simulink model "hip_controller_2026_02_23"  (R2024b)
settings: Solver=FixedStepAuto  StartTime=0.0  StopTime=simDuration  FixedStep=0.01  RelTol=1e-3  EnableMultiTasking=on
InitFcn:
  | breakp=[-1, -0.8, -0.6, -0.4, -0.2, -0.1, 0, 0.1, 0.2, 0.4, 0.6, 0.8, 1];
  | splinenew =[-1, -0.8, -0.6, -0.4, -0.2, -0.1, 0, 0, 0.005, 0.01, 0.015,0.02,0.025];
undefined symbols (not defined in the file or in its folder): Discrete, K, qbreak, Time
libraries: simulink x121, arduinolib x41, dspswit3 x21, ctrlSharedLib x2, dspfdesign x2, slpidlib x2
(part 3 of 7)

== system hip_controller_2026_02_23/Initialize Function/Config_R/Enter Config Mode ==
  Compare To Zero8 : simulink/Logic and Bit Operations/Compare To Zero  relop===  OutDataTypeStr=boolean
  Constant5 : Constant  Value=0x00
  Start_Config_R : arduinolib/I2C Write  I2CModule=0  Mode=Master  SlaveAddress=0x29  SlaveByteOrder=BigEndian  Direction=Transmitter  RegisterAddressMode=on  RegisterAddress=0x3D  SlaveDataType=uint8  DataLength=1  NoAck=off  RepeatedStart=off  OutputStatus=on  blockPlatform=ARDUINO
      settings: SourceProductName=Common
  Status : Outport
  wires:
  Start_Config_R/1 -> Compare To Zero8/1  "0 for success"
  Constant5/1 -> Start_Config_R/1
  Compare To Zero8/1 -> Status/1

== system hip_controller_2026_02_23/Initialize Function/Config_R/Start Fused (NDOF) Mode ==
  Enable : EnablePort
  Compare To Constant1 : simulink/Logic and Bit Operations/Compare To Constant  relop===  const=0  OutDataTypeStr=boolean
  Constant4 : Constant  Value=0x0C
  I2C Write8 : arduinolib/I2C Write  I2CModule=0  Mode=Master  SlaveAddress=0x29  SlaveByteOrder=BigEndian  Direction=Transmitter  RegisterAddressMode=on  RegisterAddress=0x3D  SlaveDataType=uint8  DataLength=1  NoAck=off  RepeatedStart=off  OutputStatus=on  blockPlatform=ARDUINO
      settings: SourceProductName=Common
  Status : Outport
  wires:
  Compare To Constant1/1 -> Status/1
  Constant4/1 -> I2C Write8/1
  I2C Write8/1 -> Compare To Constant1/1  "0: success"

== system hip_controller_2026_02_23/Initialize Function/Config_R/X=Z, Y=Y, Z=X ==
  Enable : EnablePort
  Compare To Constant : simulink/Logic and Bit Operations/Compare To Constant  relop=~=  const=hex2dec('06')  OutDataTypeStr=boolean
  Compare To Constant1 : simulink/Logic and Bit Operations/Compare To Constant  relop===  const=hex2dec('06')  OutDataTypeStr=boolean
  Enabled Subsystem : Subsystem  TreatAsAtomicUnit=on
  I2C Read : arduinolib/I2C Read  I2CModule=0  Mode=Master  SlaveAddress=0x29  SlaveByteOrder=LittleEndian  Direction=Receiver  RegisterAddressMode=on  RegisterAddress=0x41  SlaveDataType=uint8  DataLength=1  NoAck=off  RepeatedStart=off  OutputStatus=off  blockPlatform=ARDUINO  SampleTime=-1
      settings: SourceProductName=Common
  OR : Logic  Operator=OR  IconShape=distinctive  AllPortsSameDT=off  OutDataTypeStr=boolean
  Status : Outport
  wires:
  I2C Read/1 -> Compare To Constant1/1, Compare To Constant/1
  Compare To Constant1/1 -> OR/2
  Compare To Constant/1 -> Enabled Subsystem/Enable
  Enabled Subsystem/1(Status) -> OR/1
  OR/1 -> Status/1

== system hip_controller_2026_02_23/Initialize Function/Config_R/Z = -Z ==
  note: 0x01: Z = -Z
  Enable : EnablePort
  Compare To Constant : simulink/Logic and Bit Operations/Compare To Constant  relop=~=  const=hex2dec('01')  OutDataTypeStr=boolean
  Compare To Constant1 : simulink/Logic and Bit Operations/Compare To Constant  relop===  const=hex2dec('01')  OutDataTypeStr=boolean
  OR : Logic  Operator=OR  IconShape=distinctive  AllPortsSameDT=off  OutDataTypeStr=boolean
  Read : arduinolib/I2C Read  I2CModule=0  Mode=Master  SlaveAddress=0x29  SlaveByteOrder=LittleEndian  Direction=Receiver  RegisterAddressMode=on  RegisterAddress=0x42  SlaveDataType=uint8  DataLength=1  NoAck=off  RepeatedStart=off  OutputStatus=off  blockPlatform=ARDUINO  SampleTime=-1
      settings: SourceProductName=Common
  Write : Subsystem  TreatAsAtomicUnit=on
  Status : Outport
  wires:
  Write/1(Status) -> OR/1
  Compare To Constant/1 -> Write/Enable
  Read/1 -> Compare To Constant1/1, Compare To Constant/1
  Compare To Constant1/1 -> OR/2
  OR/1 -> Status/1

== system hip_controller_2026_02_23/LEFT LEG1/Pos and Vel normalized/Subsystem ==
  Angle : Inport
  Trigger : TriggerPort  VariantControl=Variant  PortDimensions=1
  Angle_min : Outport
  wires:
  Angle/1 -> Angle_min/1

== system hip_controller_2026_02_23/LEFT LEG1/Pos and Vel normalized/Subsystem1 ==
  Velocity : Inport
  Trigger : TriggerPort  VariantControl=Variant  PortDimensions=1
  Vel_max : Outport
  wires:
  Velocity/1 -> Vel_max/1

== system hip_controller_2026_02_23/LEFT LEG1/Pos and Vel normalized/Subsystem2 ==
  angle : Inport
  Trigger : TriggerPort  VariantControl=Variant  PortDimensions=1
  Angle_max : Outport
  wires:
  angle/1 -> Angle_max/1

== system hip_controller_2026_02_23/LEFT LEG1/Pos and Vel normalized/Subsystem3 ==
  Velocity : Inport
  Trigger : TriggerPort  VariantControl=Variant  PortDimensions=1
  Vel_min : Outport
  wires:
  Velocity/1 -> Vel_min/1

== system hip_controller_2026_02_23/LEFT LEG1/Pos and Vel normalized/Subsystem4 ==
  Clock : Inport
  angle : Inport  Port=2
  Trigger : TriggerPort  VariantControl=Variant  PortDimensions=1
  If : If  ShowElse=off
  If Action Subsystem : Subsystem  TreatAsAtomicUnit=on
  Angle_max : Outport
  wires:
  If/1 -> If Action Subsystem/Action
  angle/1 -> If Action Subsystem/2(angle), If/1
  If Action Subsystem/1(Angle_max) -> Angle_max/1  "angle_max"
  Clock/1 -> If Action Subsystem/1(Clock)  "clock"

== system hip_controller_2026_02_23/LEFT LEG1/Pos and Vel normalized/Subsystem5 ==
  Angle : Inport
  Clock : Inport  Port=2
  Trigger : TriggerPort  VariantControl=Variant  PortDimensions=1
  If : If  IfExpression=u1 < 0  ShowElse=off
  If Action Subsystem : Subsystem  TreatAsAtomicUnit=on
  Angle_min : Outport
  wires:
  If/1 -> If Action Subsystem/Action
  Angle/1 -> If Action Subsystem/1(Angle), If/1
  If Action Subsystem/1(Angle_min) -> Angle_min/1  "angle_min"
  Clock/1 -> If Action Subsystem/2(Clock)  "clock"

== system hip_controller_2026_02_23/LEFT LEG1/Pos and Vel normalized/Subsystem6 ==
  Velocity : Inport
  Clock : Inport  Port=2
  Trigger : TriggerPort  VariantControl=Variant  PortDimensions=1
  If : If  IfExpression=u1 < 0  ShowElse=off
  If Action Subsystem : Subsystem  TreatAsAtomicUnit=on
  Vel_min : Outport
  wires:
  If Action Subsystem/1(Vel_min) -> Vel_min/1  "vel_min"
  If/1 -> If Action Subsystem/Action
  Velocity/1 -> If Action Subsystem/1(Velocity), If/1
  Clock/1 -> If Action Subsystem/2(Clock)  "clock"

== system hip_controller_2026_02_23/LEFT LEG1/Pos and Vel normalized/Subsystem7 ==
  Velocity : Inport
  Clock : Inport  Port=2
  Trigger : TriggerPort  VariantControl=Variant  PortDimensions=1
  If : If  ShowElse=off
  If Action Subsystem : Subsystem  TreatAsAtomicUnit=on
  Vel_max : Outport
  wires:
  If/1 -> If Action Subsystem/Action
  Velocity/1 -> If Action Subsystem/1(Velocity), If/1
  Clock/1 -> If Action Subsystem/2(Clock)  "clock"
  If Action Subsystem/1(Vel_max) -> Vel_max/1  "vel_max"

== system hip_controller_2026_02_23/LEFT LEG3/GAIT PHASE BLOCK/CENTERING AND NORMALIZING ==
  Angle max : Inport
  Angle min : Inport  Port=2
  Vel max : Inport  Port=3
  Vel min : Inport  Port=4
  Trigger : TriggerPort  VariantControl=(inherit)  PortDimensions=1
  Abs : Abs  SaturateOnIntegerOverflow=off
  Abs1 : Abs  SaturateOnIntegerOverflow=off
  Constant : Constant  Value=0.5
  Constant1 : Constant  Value=0.5
  Divide : Product  Inputs=/*
  Product : Product
  Product1 : Product
  Sum : Sum
  Sum1 : Sum
  Sum2 : Sum  Inputs=+-
  Sum3 : Sum  Inputs=+-
  Switch : Switch  Criteria=u2 > Threshold  SaturateOnIntegerOverflow=off  InputSameDT=off
  Center vel : Outport
  Center angle : Outport  Port=2
  Gamma : Outport  Port=3
  wires:
  Divide/1 -> Gamma/1
  Abs1/1 -> Switch/3, Divide/2
  Switch/1 -> Divide/1
  Abs/1 -> Switch/1, Switch/2
  Sum3/1 -> Abs1/1
  Sum2/1 -> Abs/1
  Product1/1 -> Center vel/1
  Vel min/1 -> Sum1/2, Sum3/2
  Vel max/1 -> Sum1/1, Sum3/1
  Sum1/1 -> Product1/1
  Constant1/1 -> Product1/2
  Product/1 -> Center angle/1
  Constant/1 -> Product/2
  Sum/1 -> Product/1
  Angle min/1 -> Sum/2, Sum2/2
  Angle max/1 -> Sum/1, Sum2/1

== system hip_controller_2026_02_23/LEFT LEG3/GAIT PHASE BLOCK/LOGIC FOR THE BEGINNING ==
  Enable : EnablePort
  Constant : Constant  Value=0
  Phase to zero : Outport
  wires:
  Constant/1 -> Phase to zero/1

== system hip_controller_2026_02_23/LEFT LEG3/GAIT PHASE BLOCK/STRIDE EVENT DETECTOR ==
  In1 : Inport
  angle : Inport  Port=2
  Enable : EnablePort
  AND : Logic  IconShape=distinctive  AllPortsSameDT=off  OutDataTypeStr=boolean
  Hit Crossing5 : HitCross  HitCrossingOffset=-0.1  HitCrossingDirection=falling
  Relational Operator : RelationalOperator  OutDataTypeStr=boolean  RndMeth=Simplest  InputSameDT=off
  ~5 degrees : Constant  Value=0.08
  Out1 : Outport
  wires:
  Hit Crossing5/1 -> Out1/1
  ~5 degrees/1 -> Relational Operator/2
  Relational Operator/1 -> AND/2
  angle/1 -> Relational Operator/1
  In1/1 -> Hit Crossing5/1

== system hip_controller_2026_02_23/LEFT LEG3/GAIT PHASE BLOCK/Subsystem ==
  Input : Inport
  Trigger : TriggerPort  VariantControl=Variant  PortDimensions=1
  Angle min : Outport
  wires:
  Input/1 -> Angle min/1

== system hip_controller_2026_02_23/LEFT LEG3/GAIT PHASE BLOCK/Subsystem2 ==
  Input : Inport
  Trigger : TriggerPort  VariantControl=Variant  PortDimensions=1
  Angle max : Outport
  wires:
  Input/1 -> Angle max/1

== system hip_controller_2026_02_23/LEFT LEG3/GAIT PHASE BLOCK/Subsystem4 ==
  Input : Inport
  Trigger : TriggerPort  VariantControl=Variant  PortDimensions=1
  Vel min : Outport
  wires:
  Input/1 -> Vel min/1

== system hip_controller_2026_02_23/LEFT LEG3/GAIT PHASE BLOCK/Subsystem5 ==
  Input : Inport
  Trigger : TriggerPort  VariantControl=Variant  PortDimensions=1
  Vel max : Outport
  wires:
  Input/1 -> Vel max/1

== system hip_controller_2026_02_23/LEFT LEG3/Subsystem/SIGMOID SCALING ==
  note: a^n / (a^n + 1)
      |
      | The higher n, the more low amplitudes are scaled down
  PORTRAIT RADIUS : Inport
  Sigmoid Power : Inport  Port=2
  Constant2 : Constant
  Divide : Product  Inputs=*/
  Power : Math  Operator=pow
  Scale to 1 : Saturate  UpperLimit=1  LowerLimit=0
  Sum1 : Sum
  Out1 : Outport
  wires:
  Divide/1 -> Scale to 1/1
  PORTRAIT RADIUS/1 -> Power/1
  Power/1 -> Sum1/1, Divide/1
  Scale to 1/1 -> Out1/1
  Constant2/1 -> Sum1/2
  Sigmoid Power/1 -> Power/2  "sig_power_L"
  Sum1/1 -> Divide/2

== system hip_controller_2026_02_23/RIGHT LEG2/GAIT PHASE BLOCK/CENTERING AND NORMALIZING ==
  Angle max : Inport
  Angle min : Inport  Port=2
  Vel max : Inport  Port=3
  Vel min : Inport  Port=4
  Trigger : TriggerPort  VariantControl=(inherit)  PortDimensions=1
  Abs : Abs  SaturateOnIntegerOverflow=off
  Abs1 : Abs  SaturateOnIntegerOverflow=off
  Constant : Constant  Value=0.5
  Constant1 : Constant  Value=0.5
  Divide : Product  Inputs=/*
  Product : Product
  Product1 : Product
  Sum : Sum
  Sum1 : Sum
  Sum2 : Sum  Inputs=+-
  Sum3 : Sum  Inputs=+-
  Switch : Switch  Criteria=u2 > Threshold  SaturateOnIntegerOverflow=off  InputSameDT=off
  Center vel : Outport
  Center angle : Outport  Port=2
  Gamma : Outport  Port=3
  wires:
  Divide/1 -> Gamma/1
  Abs1/1 -> Switch/3, Divide/2
  Switch/1 -> Divide/1
  Abs/1 -> Switch/1, Switch/2
  Sum3/1 -> Abs1/1
  Sum2/1 -> Abs/1
  Product1/1 -> Center vel/1
  Vel min/1 -> Sum1/2, Sum3/2
  Vel max/1 -> Sum1/1, Sum3/1
  Sum1/1 -> Product1/1
  Constant1/1 -> Product1/2
  Product/1 -> Center angle/1
  Constant/1 -> Product/2
  Sum/1 -> Product/1
  Angle min/1 -> Sum/2, Sum2/2
  Angle max/1 -> Sum/1, Sum2/1

== system hip_controller_2026_02_23/RIGHT LEG2/GAIT PHASE BLOCK/LOGIC FOR THE BEGINNING ==
  Enable : EnablePort
  Constant : Constant  Value=0
  Phase to zero : Outport
  wires:
  Constant/1 -> Phase to zero/1

== system hip_controller_2026_02_23/RIGHT LEG2/GAIT PHASE BLOCK/STRIDE EVENT DETECTOR ==
  In1 : Inport
  angle : Inport  Port=2
  Enable : EnablePort
  AND : Logic  IconShape=distinctive  AllPortsSameDT=off  OutDataTypeStr=boolean
  Hit Crossing5 : HitCross  HitCrossingOffset=-0.1  HitCrossingDirection=falling
  Relational Operator : RelationalOperator  OutDataTypeStr=boolean  RndMeth=Simplest  InputSameDT=off
  ~5 degrees : Constant  Value=0.08
  Out1 : Outport
  wires:
  Hit Crossing5/1 -> Out1/1
  ~5 degrees/1 -> Relational Operator/2
  Relational Operator/1 -> AND/2
  angle/1 -> Relational Operator/1
  In1/1 -> Hit Crossing5/1

== system hip_controller_2026_02_23/RIGHT LEG2/GAIT PHASE BLOCK/Subsystem ==
  Input : Inport
  Trigger : TriggerPort  VariantControl=Variant  PortDimensions=1
  Angle min : Outport
  wires:
  Input/1 -> Angle min/1

== system hip_controller_2026_02_23/RIGHT LEG2/GAIT PHASE BLOCK/Subsystem2 ==
  Input : Inport
  Trigger : TriggerPort  VariantControl=Variant  PortDimensions=1
  Angle max : Outport
  wires:
  Input/1 -> Angle max/1

== system hip_controller_2026_02_23/RIGHT LEG2/GAIT PHASE BLOCK/Subsystem4 ==
  Input : Inport
  Trigger : TriggerPort  VariantControl=Variant  PortDimensions=1
  Vel min : Outport
  wires:
  Input/1 -> Vel min/1

== system hip_controller_2026_02_23/RIGHT LEG2/GAIT PHASE BLOCK/Subsystem5 ==
  Input : Inport
  Trigger : TriggerPort  VariantControl=Variant  PortDimensions=1
  Vel max : Outport
  wires:
  Input/1 -> Vel max/1

== system hip_controller_2026_02_23/RIGHT LEG2/Subsystem/SIGMOID SCALING ==
  note: a^n / (a^n + 1)
      |
      | The higher n, the more low amplitudes are scaled down
  PORTRAIT RADIUS : Inport
  sigmoid_power : Inport  Port=2
  Constant2 : Constant
  Divide : Product  Inputs=*/
  Power : Math  Operator=pow
  Scale to 1 : Saturate  UpperLimit=1  LowerLimit=0
  Sum1 : Sum
  Out1 : Outport
  wires:
  Divide/1 -> Scale to 1/1
  PORTRAIT RADIUS/1 -> Power/1
  Power/1 -> Sum1/1, Divide/1
  Scale to 1/1 -> Out1/1
  Constant2/1 -> Sum1/2
  sigmoid_power/1 -> Power/2
  Sum1/1 -> Divide/2

== system hip_controller_2026_02_23/RIGHT_LEG1/Pos and Vel normalized/Subsystem ==
  Angle : Inport
  Trigger : TriggerPort  VariantControl=Variant  PortDimensions=1
  Angle_min : Outport
  wires:
  Angle/1 -> Angle_min/1

== system hip_controller_2026_02_23/RIGHT_LEG1/Pos and Vel normalized/Subsystem1 ==
  Velocity : Inport
  Trigger : TriggerPort  VariantControl=Variant  PortDimensions=1
  Vel_max : Outport
  wires:
  Velocity/1 -> Vel_max/1

== system hip_controller_2026_02_23/RIGHT_LEG1/Pos and Vel normalized/Subsystem2 ==
  angle : Inport
  Trigger : TriggerPort  VariantControl=Variant  PortDimensions=1
  Angle_max : Outport
  wires:
  angle/1 -> Angle_max/1

== system hip_controller_2026_02_23/RIGHT_LEG1/Pos and Vel normalized/Subsystem3 ==
  Velocity : Inport
  Trigger : TriggerPort  VariantControl=Variant  PortDimensions=1
  Vel_min : Outport
  wires:
  Velocity/1 -> Vel_min/1

== system hip_controller_2026_02_23/RIGHT_LEG1/Pos and Vel normalized/Subsystem4 ==
  Clock : Inport
  angle : Inport  Port=2
  Trigger : TriggerPort  VariantControl=Variant  PortDimensions=1
  If : If  ShowElse=off
  If Action Subsystem : Subsystem  TreatAsAtomicUnit=on
  Angle_max : Outport
  wires:
  If/1 -> If Action Subsystem/Action
  angle/1 -> If Action Subsystem/2(angle), If/1
  If Action Subsystem/1(Angle_max) -> Angle_max/1  "angle_max"
  Clock/1 -> If Action Subsystem/1(Clock)  "clock"

== system hip_controller_2026_02_23/RIGHT_LEG1/Pos and Vel normalized/Subsystem5 ==
  Angle : Inport
  Clock : Inport  Port=2
  Trigger : TriggerPort  VariantControl=Variant  PortDimensions=1
  If : If  IfExpression=u1 < 0  ShowElse=off
  If Action Subsystem : Subsystem  TreatAsAtomicUnit=on
  Angle_min : Outport
  wires:
  If/1 -> If Action Subsystem/Action
  Angle/1 -> If Action Subsystem/1(Angle), If/1
  If Action Subsystem/1(Angle_min) -> Angle_min/1  "angle_min"
  Clock/1 -> If Action Subsystem/2(Clock)  "clock"

== system hip_controller_2026_02_23/RIGHT_LEG1/Pos and Vel normalized/Subsystem6 ==
  Velocity : Inport
  Clock : Inport  Port=2
  Trigger : TriggerPort  VariantControl=Variant  PortDimensions=1
  If : If  IfExpression=u1 < 0  ShowElse=off
  If Action Subsystem : Subsystem  TreatAsAtomicUnit=on
  Vel_min : Outport
  wires:
  If Action Subsystem/1(Vel_min) -> Vel_min/1  "vel_min"
  If/1 -> If Action Subsystem/Action
  Velocity/1 -> If Action Subsystem/1(Velocity), If/1
  Clock/1 -> If Action Subsystem/2(Clock)  "clock"

== system hip_controller_2026_02_23/RIGHT_LEG1/Pos and Vel normalized/Subsystem7 ==
  Velocity : Inport
  Clock : Inport  Port=2
  Trigger : TriggerPort  VariantControl=Variant  PortDimensions=1
  If : If  ShowElse=off
  If Action Subsystem : Subsystem  TreatAsAtomicUnit=on
  Vel_max : Outport
  wires:
  If/1 -> If Action Subsystem/Action
  Velocity/1 -> If Action Subsystem/1(Velocity), If/1
  Clock/1 -> If Action Subsystem/2(Clock)  "clock"
  If Action Subsystem/1(Vel_max) -> Vel_max/1  "vel_max"

== system hip_controller_2026_02_23/Subsystem3/Left Motor Velocity/Motor Actual Position Receive ==
  SWITCH : Inport
  Bus Selector1 : BusSelector  OutputSignals=Data
  CAN Receive : arduinolib/CAN Receive  Priority=4  outputDataType=CAN Msg  identifierType=Standard (11-bit identifier)  messageId=0  msgLength=8  SampleTime=0.01  outputError=off  outputRemote=off
      settings: SourceProductName=Common
  CHINESE CORRECTION : Subsystem
  Constant1 : Constant  Value=0
  Constant3 : Constant
  Data Type Conversion2 : DataTypeConversion  OutDataTypeStr=uint16  SaturateOnIntegerOverflow=off  RndMeth=Floor
  Delay : Delay  DelayLength=1
  Delay2 : Delay
  Memory2 : Memory
  N-Sample Switch2 : dspswit3/N-Sample Switch  N=10  reset=on  TriggerType=Rising edge  Ts=0.01
  Sum : Sum  Inputs=-|+
  Switch2 : Switch  Criteria=u2 > Threshold  SaturateOnIntegerOverflow=off  InputSameDT=off
  Terminator1 : Terminator
  Unpack2 : Subsystem
  Zero-Order Hold1 : ZeroOrderHold  SampleTime=0.01
  MOTOR POSITION : Outport
  MOTOR SPEED : Outport  Port=2
  MOTOR TORQUE : Outport  Port=3
  wires:
  Switch2/1 -> Sum/1, Delay2/1
  CAN Receive/1 -> Bus Selector1/1
  SWITCH/1 -> Zero-Order Hold1/1
  N-Sample Switch2/1 -> Switch2/2
  Memory2/1 -> Switch2/1
  Constant1/1 -> N-Sample Switch2/1
  Sum/1 -> Delay/1
  Unpack2/2(speed) -> MOTOR SPEED/1  "MOTOR SPEED"
  Delay2/1 -> Memory2/1
  Bus Selector1/1 -> Data Type Conversion2/1  "<Data>"
  CHINESE CORRECTION/1(Out1) -> Sum/2, Switch2/3
  Constant3/1 -> N-Sample Switch2/2
  Unpack2/1(position) -> CHINESE CORRECTION/1(position)  "MOTOR POS"
  Data Type Conversion2/1 -> Unpack2/1(Data)
  CAN Receive/2 -> Terminator1/1
  Delay/1 -> MOTOR POSITION/1
  Unpack2/3(torque) -> MOTOR TORQUE/1  "MOTOR TORQUE"
  Zero-Order Hold1/1 -> N-Sample Switch2/3, CHINESE CORRECTION/Enable

== system hip_controller_2026_02_23/Subsystem3/Left Motor Velocity/Subsystem ==
  Motor command : Inport
  SWITCH : Inport  Port=2
  CAN Pack1 : Subsystem
  CAN Transmit1 : arduinolib/CAN Transmit  Priority=3  inputDataType=Raw data  BlockingMode_=on  BlockTimeout_=1  outputStatus=off  identifierType=Standard (11-bit identifier)  messageId=3  msgLength=8  remoteFrame=off
      settings: SourceProductName=Common
  Constant7 : Constant  Value=0  OutDataTypeStr=single  SampleTime=0.01
  DISABLE1 : Constant  Value=269.7/18  OutDataTypeStr=single
  Data Type Conversion3 : DataTypeConversion  OutDataTypeStr=single  SaturateOnIntegerOverflow=off  RndMeth=Floor
  Demux1 : Demux  Outputs=5
  ENABLE1 : Constant  Value=14.975  OutDataTypeStr=single
  IsNaN : RelationalOperator  Operator=isNaN  OutDataTypeStr=boolean  RndMeth=Simplest  InputSameDT=off
  N-Sample Switch4 : dspswit3/N-Sample Switch  N=15  reset=on  TriggerType=Either edge  Ts=0.01
  Rate Transition : RateTransition  OutPortSampleTime=0.01
  Subsystem2 : Subsystem
  Switch : Switch  Criteria=u2 > Threshold  SaturateOnIntegerOverflow=off  InputSameDT=off
  Switch3 : Switch  Criteria=u2 > Threshold  SaturateOnIntegerOverflow=off  InputSameDT=off
  wires:
  Demux1/4 -> CAN Pack1/4(Kd)
  Data Type Conversion3/1 -> Subsystem2/2(Velocity)
  Switch3/1 -> Subsystem2/1(Enable)
  Demux1/1 -> CAN Pack1/1(Position)
  Motor command/1 -> Data Type Conversion3/1, IsNaN/1
  Demux1/5 -> CAN Pack1/5(Torque)
  ENABLE1/1 -> Switch3/1
  Demux1/2 -> CAN Pack1/2(Velocity)
  Rate Transition/1 -> N-Sample Switch4/3
  IsNaN/1 -> Switch/2
  DISABLE1/1 -> Switch3/3
  Subsystem2/1(Enter_motor_mode) -> N-Sample Switch4/1
  Demux1/3 -> CAN Pack1/3(Kp)
  N-Sample Switch4/1 -> Demux1/1
  Switch/1 -> Rate Transition/1, Switch3/2
  CAN Pack1/1(CAN Data) -> CAN Transmit1/1
  Subsystem2/2(Velocity_value) -> N-Sample Switch4/2
  Constant7/1 -> Switch/1
  SWITCH/1 -> Switch/3

== system hip_controller_2026_02_23/Subsystem3/Right Motor Velocity/Motor Actual Position Receive ==
  SWITCH : Inport
  Bus Selector1 : BusSelector  OutputSignals=Data
  CAN Receive : arduinolib/CAN Receive  Priority=2  outputDataType=CAN Msg  identifierType=Standard (11-bit identifier)  messageId=0  msgLength=8  SampleTime=0.01  outputError=off  outputRemote=off
      settings: SourceProductName=Common
  CHINESE CORRECTION : Subsystem
  Constant1 : Constant  Value=0
  Constant3 : Constant
  Data Type Conversion2 : DataTypeConversion  OutDataTypeStr=uint16  SaturateOnIntegerOverflow=off  RndMeth=Floor
  Delay : Delay  DelayLength=1
  Delay2 : Delay
  Memory2 : Memory
  N-Sample Switch2 : dspswit3/N-Sample Switch  N=10  reset=on  TriggerType=Rising edge  Ts=0.01
  Sum : Sum  Inputs=-|+
  Switch2 : Switch  Criteria=u2 > Threshold  SaturateOnIntegerOverflow=off  InputSameDT=off
  Terminator1 : Terminator
  Unpack2 : Subsystem
  Zero-Order Hold1 : ZeroOrderHold  SampleTime=0.01
  MOTOR POSITION : Outport
  MOTOR SPEED : Outport  Port=2
  MOTOR TORQUE : Outport  Port=3
  wires:
  Switch2/1 -> Sum/1, Delay2/1
  CAN Receive/1 -> Bus Selector1/1
  SWITCH/1 -> Zero-Order Hold1/1
  N-Sample Switch2/1 -> Switch2/2
  Memory2/1 -> Switch2/1
  Constant1/1 -> N-Sample Switch2/1
  Sum/1 -> Delay/1
  Unpack2/2(speed) -> MOTOR SPEED/1  "MOTOR SPEED"
  Delay2/1 -> Memory2/1
  Bus Selector1/1 -> Data Type Conversion2/1  "<Data>"
  CHINESE CORRECTION/1(Out1) -> Sum/2, Switch2/3
  Constant3/1 -> N-Sample Switch2/2
  Unpack2/1(position) -> CHINESE CORRECTION/1(position)  "MOTOR POS"
  Data Type Conversion2/1 -> Unpack2/1(Data)
  CAN Receive/2 -> Terminator1/1
  Delay/1 -> MOTOR POSITION/1
  Unpack2/3(torque) -> MOTOR TORQUE/1  "MOTOR TORQUE"
  Zero-Order Hold1/1 -> N-Sample Switch2/3, CHINESE CORRECTION/Enable

== system hip_controller_2026_02_23/Subsystem3/Right Motor Velocity/Subsystem ==
  Motor command : Inport
  SWITCH : Inport  Port=2
  CAN Pack1 : Subsystem
  CAN Transmit1 : arduinolib/CAN Transmit  Priority=1  inputDataType=Raw data  BlockingMode_=on  BlockTimeout_=1  outputStatus=off  identifierType=Standard (11-bit identifier)  messageId=4  msgLength=8  remoteFrame=off
      settings: SourceProductName=Common
  Constant7 : Constant  Value=0  OutDataTypeStr=single  SampleTime=0.01
  DISABLE1 : Constant  Value=269.7/18  OutDataTypeStr=single
  Data Type Conversion3 : DataTypeConversion  OutDataTypeStr=single  SaturateOnIntegerOverflow=off  RndMeth=Floor
  Demux1 : Demux  Outputs=5
  ENABLE1 : Constant  Value=14.975  OutDataTypeStr=single
  IsNaN : RelationalOperator  Operator=isNaN  OutDataTypeStr=boolean  RndMeth=Simplest  InputSameDT=off
  N-Sample Switch4 : dspswit3/N-Sample Switch  N=15  reset=on  TriggerType=Either edge  Ts=0.01
  Rate Transition : RateTransition  OutPortSampleTime=0.01
  Subsystem2 : Subsystem
  Switch : Switch  Criteria=u2 > Threshold  SaturateOnIntegerOverflow=off  InputSameDT=off
  Switch3 : Switch  Criteria=u2 > Threshold  SaturateOnIntegerOverflow=off  InputSameDT=off
  wires:
  Demux1/4 -> CAN Pack1/4(Kd)
  Data Type Conversion3/1 -> Subsystem2/2(Velocity)
  Switch3/1 -> Subsystem2/1(Enable)
  Demux1/1 -> CAN Pack1/1(Position)
  Motor command/1 -> Data Type Conversion3/1, IsNaN/1
  Demux1/5 -> CAN Pack1/5(Torque)
  ENABLE1/1 -> Switch3/1
  Demux1/2 -> CAN Pack1/2(Velocity)
  Rate Transition/1 -> N-Sample Switch4/3
  IsNaN/1 -> Switch/2
  DISABLE1/1 -> Switch3/3
  Subsystem2/1(Enter_motor_mode) -> N-Sample Switch4/1
  Demux1/3 -> CAN Pack1/3(Kp)
  N-Sample Switch4/1 -> Demux1/1
  Switch/1 -> Rate Transition/1, Switch3/2
  CAN Pack1/1(CAN Data) -> CAN Transmit1/1
  Subsystem2/2(Velocity_value) -> N-Sample Switch4/2
  Constant7/1 -> Switch/1
  SWITCH/1 -> Switch/3

== system hip_controller_2026_02_23/Subsystem4/Left Motor Velocity/Motor Actual Position Receive ==
  SWITCH : Inport
  Bus Selector1 : BusSelector  OutputSignals=Data
  CAN Receive : arduinolib/CAN Receive  Priority=4  outputDataType=CAN Msg  identifierType=Standard (11-bit identifier)  messageId=0  msgLength=8  SampleTime=0.01  outputError=off  outputRemote=off
      settings: SourceProductName=Common
  CHINESE CORRECTION : Subsystem
  Constant1 : Constant  Value=0
  Constant3 : Constant
  Data Type Conversion2 : DataTypeConversion  OutDataTypeStr=uint16  SaturateOnIntegerOverflow=off  RndMeth=Floor
  Delay : Delay  DelayLength=1
  Delay2 : Delay
  Memory2 : Memory
  N-Sample Switch2 : dspswit3/N-Sample Switch  N=10  reset=on  TriggerType=Rising edge  Ts=0.01
  Sum : Sum  Inputs=-|+
  Switch2 : Switch  Criteria=u2 > Threshold  SaturateOnIntegerOverflow=off  InputSameDT=off
  Terminator1 : Terminator
  Unpack2 : Subsystem
  MOTOR POSITION : Outport
  MOTOR SPEED : Outport  Port=2
  MOTOR TORQUE : Outport  Port=3
  wires:
  Switch2/1 -> Sum/1, Delay2/1
  CAN Receive/1 -> Bus Selector1/1
  SWITCH/1 -> N-Sample Switch2/3, CHINESE CORRECTION/Enable
  N-Sample Switch2/1 -> Switch2/2
  Memory2/1 -> Switch2/1
  Constant1/1 -> N-Sample Switch2/1
  Sum/1 -> Delay/1
  Unpack2/2(speed) -> MOTOR SPEED/1  "MOTOR SPEED"
  Delay2/1 -> Memory2/1
  Bus Selector1/1 -> Data Type Conversion2/1  "<Data>"
  CHINESE CORRECTION/1(Out1) -> Sum/2, Switch2/3
  Constant3/1 -> N-Sample Switch2/2
  Unpack2/1(position) -> CHINESE CORRECTION/1(position)  "MOTOR POS"
  Data Type Conversion2/1 -> Unpack2/1(Data)
  CAN Receive/2 -> Terminator1/1
  Delay/1 -> MOTOR POSITION/1
  Unpack2/3(torque) -> MOTOR TORQUE/1  "MOTOR TORQUE"

== system hip_controller_2026_02_23/Subsystem4/Left Motor Velocity/Subsystem ==
  Motor command : Inport
  SWITCH : Inport  Port=2
  CAN Pack1 : Subsystem
  CAN Transmit1 : arduinolib/CAN Transmit  Priority=3  inputDataType=Raw data  BlockingMode_=on  BlockTimeout_=1  outputStatus=off  identifierType=Standard (11-bit identifier)  messageId=3  msgLength=8  remoteFrame=off
      settings: SourceProductName=Common
  Constant7 : Constant  Value=0  OutDataTypeStr=single  SampleTime=0.01
  DISABLE1 : Constant  Value=269.7/18  OutDataTypeStr=single
  Data Type Conversion3 : DataTypeConversion  OutDataTypeStr=single  SaturateOnIntegerOverflow=off  RndMeth=Floor
  Demux1 : Demux  Outputs=5
  ENABLE1 : Constant  Value=14.975  OutDataTypeStr=single
  IsNaN : RelationalOperator  Operator=isNaN  OutDataTypeStr=boolean  RndMeth=Simplest  InputSameDT=off
  N-Sample Switch4 : dspswit3/N-Sample Switch  N=15  reset=on  TriggerType=Either edge  Ts=0.01
  Rate Transition : RateTransition  OutPortSampleTime=0.01
  Subsystem2 : Subsystem
  Switch : Switch  Criteria=u2 > Threshold  SaturateOnIntegerOverflow=off  InputSameDT=off
  Switch3 : Switch  Criteria=u2 > Threshold  SaturateOnIntegerOverflow=off  InputSameDT=off
  wires:
  Demux1/4 -> CAN Pack1/4(Kd)
  Data Type Conversion3/1 -> Subsystem2/2(Velocity)
  Switch3/1 -> Subsystem2/1(Enable)
  Demux1/1 -> CAN Pack1/1(Position)
  Motor command/1 -> Data Type Conversion3/1, IsNaN/1
  Demux1/5 -> CAN Pack1/5(Torque)
  ENABLE1/1 -> Switch3/1
  Demux1/2 -> CAN Pack1/2(Velocity)
  Rate Transition/1 -> N-Sample Switch4/3
  IsNaN/1 -> Switch/2
  DISABLE1/1 -> Switch3/3
  Subsystem2/1(Enter_motor_mode) -> N-Sample Switch4/1
  Demux1/3 -> CAN Pack1/3(Kp)
  N-Sample Switch4/1 -> Demux1/1
  Switch/1 -> Rate Transition/1, Switch3/2
  CAN Pack1/1(CAN Data) -> CAN Transmit1/1
  Subsystem2/2(Velocity_value) -> N-Sample Switch4/2
  Constant7/1 -> Switch/1
  SWITCH/1 -> Switch/3

== system hip_controller_2026_02_23/Subsystem4/PID3/Subsystem2 ==
  x : Inport
  Constant : Constant  Value=2
  Integrator1 : Integrator  InitialConditionSource=external
  Integrator2 : Integrator
  Product : Product  RndMeth=Zero
  Product1 : Product  RndMeth=Zero
  Product2 : Product  Inputs=3  RndMeth=Zero
  Sum : Sum  Inputs=|+-
  Sum1 : Sum  Inputs=|+-
  wn : Constant  Value=wn
  x0 : Constant  Value=x0
  zt : Constant  Value=zt
  y : Outport  VectorParamsAs1DForOutWhenUnconnected=off
  yd : Outport  Port=2  VectorParamsAs1DForOutWhenUnconnected=off
  wires:
  Sum/1 -> Product/2
  wn/1 -> Product/1, Product1/1
  Sum1/1 -> Sum/1
  x0/1 -> Integrator1/2
  Integrator2/1 -> Product1/2, Product2/1
  Product/1 -> Integrator2/1
  x/1 -> Sum1/1
  Product1/1 -> Integrator1/1, yd/1
  Integrator1/1 -> Sum1/2, y/1
  Product2/1 -> Sum/2
  zt/1 -> Product2/3
  Constant/1 -> Product2/2

== system hip_controller_2026_02_23/Subsystem4/PID4/Subsystem2 ==
  x : Inport
  Constant : Constant  Value=2
  Integrator1 : Integrator  InitialConditionSource=external
  Integrator2 : Integrator
  Product : Product  RndMeth=Zero
  Product1 : Product  RndMeth=Zero
  Product2 : Product  Inputs=3  RndMeth=Zero
  Sum : Sum  Inputs=|+-
  Sum1 : Sum  Inputs=|+-
  wn : Constant  Value=wn
  x0 : Constant  Value=x0
  zt : Constant  Value=zt
  y : Outport  VectorParamsAs1DForOutWhenUnconnected=off
  yd : Outport  Port=2  VectorParamsAs1DForOutWhenUnconnected=off
  wires:
  Sum/1 -> Product/2
  wn/1 -> Product/1, Product1/1
  Sum1/1 -> Sum/1
  x0/1 -> Integrator1/2
  Integrator2/1 -> Product1/2, Product2/1
  Product/1 -> Integrator2/1
  x/1 -> Sum1/1
  Product1/1 -> Integrator1/1, yd/1
  Integrator1/1 -> Sum1/2, y/1
  Product2/1 -> Sum/2
  zt/1 -> Product2/3
  Constant/1 -> Product2/2

== system hip_controller_2026_02_23/Subsystem4/Right Motor Velocity/Motor Actual Position Receive ==
  SWITCH : Inport
  Bus Selector1 : BusSelector  OutputSignals=Data
  CAN Receive : arduinolib/CAN Receive  Priority=2  outputDataType=CAN Msg  identifierType=Standard (11-bit identifier)  messageId=0  msgLength=8  SampleTime=0.01  outputError=off  outputRemote=off
      settings: SourceProductName=Common
  CHINESE CORRECTION : Subsystem
  Constant1 : Constant  Value=0
  Constant3 : Constant
  Data Type Conversion2 : DataTypeConversion  OutDataTypeStr=uint16  SaturateOnIntegerOverflow=off  RndMeth=Floor
  Delay : Delay  DelayLength=1
  Delay2 : Delay
  Memory2 : Memory
  N-Sample Switch2 : dspswit3/N-Sample Switch  N=10  reset=on  TriggerType=Rising edge  Ts=0.01
  Sum : Sum  Inputs=-|+
  Switch2 : Switch  Criteria=u2 > Threshold  SaturateOnIntegerOverflow=off  InputSameDT=off
  Terminator1 : Terminator
  Unpack2 : Subsystem
  MOTOR POSITION : Outport
  MOTOR SPEED : Outport  Port=2
  MOTOR TORQUE : Outport  Port=3
  wires:
  Switch2/1 -> Sum/1, Delay2/1
  CAN Receive/1 -> Bus Selector1/1
  SWITCH/1 -> N-Sample Switch2/3, CHINESE CORRECTION/Enable
  N-Sample Switch2/1 -> Switch2/2
  Memory2/1 -> Switch2/1
  Constant1/1 -> N-Sample Switch2/1
  Sum/1 -> Delay/1
  Unpack2/2(speed) -> MOTOR SPEED/1  "MOTOR SPEED"
  Delay2/1 -> Memory2/1
  Bus Selector1/1 -> Data Type Conversion2/1  "<Data>"
  CHINESE CORRECTION/1(Out1) -> Sum/2, Switch2/3
  Constant3/1 -> N-Sample Switch2/2
  Unpack2/1(position) -> CHINESE CORRECTION/1(position)  "MOTOR POS"
  Data Type Conversion2/1 -> Unpack2/1(Data)
  CAN Receive/2 -> Terminator1/1
  Delay/1 -> MOTOR POSITION/1
  Unpack2/3(torque) -> MOTOR TORQUE/1  "MOTOR TORQUE"

== system hip_controller_2026_02_23/Subsystem4/Right Motor Velocity/Subsystem ==
  Motor command : Inport
  SWITCH : Inport  Port=2
  CAN Pack1 : Subsystem
  CAN Transmit1 : arduinolib/CAN Transmit  Priority=1  inputDataType=Raw data  BlockingMode_=on  BlockTimeout_=1  outputStatus=off  identifierType=Standard (11-bit identifier)  messageId=4  msgLength=8  remoteFrame=off
      settings: SourceProductName=Common
  Constant7 : Constant  Value=0  OutDataTypeStr=single  SampleTime=0.01
  DISABLE1 : Constant  Value=269.7/18  OutDataTypeStr=single
  Data Type Conversion3 : DataTypeConversion  OutDataTypeStr=single  SaturateOnIntegerOverflow=off  RndMeth=Floor
  Demux1 : Demux  Outputs=5
  ENABLE1 : Constant  Value=14.975  OutDataTypeStr=single
  IsNaN : RelationalOperator  Operator=isNaN  OutDataTypeStr=boolean  RndMeth=Simplest  InputSameDT=off
  N-Sample Switch4 : dspswit3/N-Sample Switch  N=15  reset=on  TriggerType=Either edge  Ts=0.01
  Rate Transition : RateTransition  OutPortSampleTime=0.01
  Subsystem2 : Subsystem
  Switch : Switch  Criteria=u2 > Threshold  SaturateOnIntegerOverflow=off  InputSameDT=off
  Switch3 : Switch  Criteria=u2 > Threshold  SaturateOnIntegerOverflow=off  InputSameDT=off
  wires:
  Demux1/4 -> CAN Pack1/4(Kd)
  Data Type Conversion3/1 -> Subsystem2/2(Velocity)
  Switch3/1 -> Subsystem2/1(Enable)
  Demux1/1 -> CAN Pack1/1(Position)
  Motor command/1 -> Data Type Conversion3/1, IsNaN/1
  Demux1/5 -> CAN Pack1/5(Torque)
  ENABLE1/1 -> Switch3/1
  Demux1/2 -> CAN Pack1/2(Velocity)
  Rate Transition/1 -> N-Sample Switch4/3
  IsNaN/1 -> Switch/2
  DISABLE1/1 -> Switch3/3
  Subsystem2/1(Enter_motor_mode) -> N-Sample Switch4/1
  Demux1/3 -> CAN Pack1/3(Kp)
  N-Sample Switch4/1 -> Demux1/1
  Switch/1 -> Rate Transition/1, Switch3/2
  CAN Pack1/1(CAN Data) -> CAN Transmit1/1
  Subsystem2/2(Velocity_value) -> N-Sample Switch4/2
  Constant7/1 -> Switch/1
  SWITCH/1 -> Switch/3

== system hip_controller_2026_02_23/Subsystem5/Left Motor Velocity1/Motor Actual Position Receive ==
  SWITCH : Inport
  Bus Selector1 : BusSelector  OutputSignals=Data
  CAN Receive : arduinolib/CAN Receive  outputDataType=CAN Msg  identifierType=Standard (11-bit identifier)  messageId=0  msgLength=8  SampleTime=0.01  outputError=off  outputRemote=off
      settings: SourceProductName=Common
  CHINESE CORRECTION : Subsystem
  Constant1 : Constant  Value=0
  Constant3 : Constant
  Data Type Conversion2 : DataTypeConversion  OutDataTypeStr=uint16  SaturateOnIntegerOverflow=off  RndMeth=Floor
  Delay : Delay  DelayLength=1
  Delay2 : Delay
  Memory2 : Memory
  N-Sample Switch2 : dspswit3/N-Sample Switch  N=10  reset=on  TriggerType=Rising edge  Ts=0.01
  Sum : Sum  Inputs=-|+
  Switch2 : Switch  Criteria=u2 > Threshold  SaturateOnIntegerOverflow=off  InputSameDT=off
  Terminator1 : Terminator
  Unpack2 : Subsystem
  MOTOR POSITION : Outport
  MOTOR SPEED : Outport  Port=2
  MOTOR TORQUE : Outport  Port=3
  wires:
  Switch2/1 -> Sum/1, Delay2/1
  CAN Receive/1 -> Bus Selector1/1
  SWITCH/1 -> N-Sample Switch2/3, CHINESE CORRECTION/Enable
  N-Sample Switch2/1 -> Switch2/2
  Memory2/1 -> Switch2/1
  Constant1/1 -> N-Sample Switch2/1
  Sum/1 -> Delay/1
  Unpack2/2(speed) -> MOTOR SPEED/1  "MOTOR SPEED"
  Delay2/1 -> Memory2/1
  Bus Selector1/1 -> Data Type Conversion2/1  "<Data>"
  CHINESE CORRECTION/1(Out1) -> Sum/2, Switch2/3
  Constant3/1 -> N-Sample Switch2/2
  Unpack2/1(position) -> CHINESE CORRECTION/1(position)  "MOTOR POS"
  Data Type Conversion2/1 -> Unpack2/1(Data)
  CAN Receive/2 -> Terminator1/1
  Delay/1 -> MOTOR POSITION/1
  Unpack2/3(torque) -> MOTOR TORQUE/1  "MOTOR TORQUE"

== system hip_controller_2026_02_23/Subsystem5/Left Motor Velocity1/Subsystem ==
  Motor command : Inport
  SWITCH : Inport  Port=2
  CAN Pack1 : Subsystem
  CAN Transmit1 : arduinolib/CAN Transmit  inputDataType=Raw data  BlockingMode_=on  BlockTimeout_=1  outputStatus=off  identifierType=Standard (11-bit identifier)  messageId=4  msgLength=8  remoteFrame=off
      settings: SourceProductName=Common
  Constant7 : Constant  Value=0  OutDataTypeStr=single  SampleTime=0.01
  DISABLE1 : Constant  Value=269.7/18  OutDataTypeStr=single
  Data Type Conversion3 : DataTypeConversion  OutDataTypeStr=single  SaturateOnIntegerOverflow=off  RndMeth=Floor
  Demux1 : Demux  Outputs=5
  ENABLE1 : Constant  Value=14.975  OutDataTypeStr=single
  IsNaN : RelationalOperator  Operator=isNaN  OutDataTypeStr=boolean  RndMeth=Simplest  InputSameDT=off
  N-Sample Switch4 : dspswit3/N-Sample Switch  N=15  reset=on  TriggerType=Either edge  Ts=0.01
  Rate Transition : RateTransition  OutPortSampleTime=0.01
  Subsystem2 : Subsystem
  Switch : Switch  Criteria=u2 > Threshold  SaturateOnIntegerOverflow=off  InputSameDT=off
  Switch3 : Switch  Criteria=u2 > Threshold  SaturateOnIntegerOverflow=off  InputSameDT=off
  wires:
  Demux1/4 -> CAN Pack1/4(Kd)
  Data Type Conversion3/1 -> Subsystem2/2(Velocity)
  Switch3/1 -> Subsystem2/1(Enable)
  Demux1/1 -> CAN Pack1/1(Position)
  Motor command/1 -> Data Type Conversion3/1, IsNaN/1
  Demux1/5 -> CAN Pack1/5(Torque)
  ENABLE1/1 -> Switch3/1
  Demux1/2 -> CAN Pack1/2(Velocity)
  Rate Transition/1 -> N-Sample Switch4/3
  IsNaN/1 -> Switch/2
  DISABLE1/1 -> Switch3/3
  Subsystem2/1(Enter_motor_mode) -> N-Sample Switch4/1
  Demux1/3 -> CAN Pack1/3(Kp)
  N-Sample Switch4/1 -> Demux1/1
  Switch/1 -> Rate Transition/1, Switch3/2
  CAN Pack1/1(CAN Data) -> CAN Transmit1/1
  Subsystem2/2(Velocity_value) -> N-Sample Switch4/2
  Constant7/1 -> Switch/1
  SWITCH/1 -> Switch/3

== system hip_controller_2026_02_23/Subsystem5/PID1/Subsystem2 ==
  x : Inport
  Constant : Constant  Value=2
  Integrator1 : Integrator  InitialConditionSource=external
  Integrator2 : Integrator
  Product : Product  RndMeth=Zero
  Product1 : Product  RndMeth=Zero
  Product2 : Product  Inputs=3  RndMeth=Zero
  Sum : Sum  Inputs=|+-
  Sum1 : Sum  Inputs=|+-
  wn : Constant  Value=wn
  x0 : Constant  Value=x0
  zt : Constant  Value=zt
  y : Outport  VectorParamsAs1DForOutWhenUnconnected=off
  yd : Outport  Port=2  VectorParamsAs1DForOutWhenUnconnected=off
  wires:
  Sum/1 -> Product/2
  wn/1 -> Product/1, Product1/1
  Sum1/1 -> Sum/1
  x0/1 -> Integrator1/2
  Integrator2/1 -> Product1/2, Product2/1
  Product/1 -> Integrator2/1
  x/1 -> Sum1/1
  Product1/1 -> Integrator1/1, yd/1
  Integrator1/1 -> Sum1/2, y/1
  Product2/1 -> Sum/2
  zt/1 -> Product2/3
  Constant/1 -> Product2/2

== system hip_controller_2026_02_23/Subsystem5/PID2/Subsystem2 ==
  x : Inport
  Constant : Constant  Value=2
  Integrator1 : Integrator  InitialConditionSource=external
  Integrator2 : Integrator
  Product : Product  RndMeth=Zero
  Product1 : Product  RndMeth=Zero
  Product2 : Product  Inputs=3  RndMeth=Zero
  Sum : Sum  Inputs=|+-
  Sum1 : Sum  Inputs=|+-
  wn : Constant  Value=wn
  x0 : Constant  Value=x0
  zt : Constant  Value=zt
  y : Outport  VectorParamsAs1DForOutWhenUnconnected=off
  yd : Outport  Port=2  VectorParamsAs1DForOutWhenUnconnected=off
  wires:
  Sum/1 -> Product/2
  wn/1 -> Product/1, Product1/1
  Sum1/1 -> Sum/1
  x0/1 -> Integrator1/2
  Integrator2/1 -> Product1/2, Product2/1
  Product/1 -> Integrator2/1
  x/1 -> Sum1/1
  Product1/1 -> Integrator1/1, yd/1
  Integrator1/1 -> Sum1/2, y/1
  Product2/1 -> Sum/2
  zt/1 -> Product2/3
  Constant/1 -> Product2/2

== system hip_controller_2026_02_23/Subsystem5/Right Motor Velocity1/Motor Actual Position Receive ==
  SWITCH : Inport
  Bus Selector1 : BusSelector  OutputSignals=Data
  CAN Receive : arduinolib/CAN Receive  outputDataType=CAN Msg  identifierType=Standard (11-bit identifier)  messageId=0  msgLength=8  SampleTime=0.01  outputError=off  outputRemote=off
      settings: SourceProductName=Common
  CHINESE CORRECTION : Subsystem
  Constant1 : Constant  Value=0
  Constant3 : Constant
  Data Type Conversion2 : DataTypeConversion  OutDataTypeStr=uint16  SaturateOnIntegerOverflow=off  RndMeth=Floor
  Delay : Delay  DelayLength=1
  Delay2 : Delay
  Memory2 : Memory
  N-Sample Switch2 : dspswit3/N-Sample Switch  N=10  reset=on  TriggerType=Rising edge  Ts=0.01
  Sum : Sum  Inputs=-|+
  Switch2 : Switch  Criteria=u2 > Threshold  SaturateOnIntegerOverflow=off  InputSameDT=off
  Terminator1 : Terminator
  Unpack2 : Subsystem
  MOTOR POSITION : Outport
  MOTOR SPEED : Outport  Port=2
  MOTOR TORQUE : Outport  Port=3
  wires:
  Switch2/1 -> Sum/1, Delay2/1
  CAN Receive/1 -> Bus Selector1/1
  SWITCH/1 -> N-Sample Switch2/3, CHINESE CORRECTION/Enable
  N-Sample Switch2/1 -> Switch2/2
  Memory2/1 -> Switch2/1
  Constant1/1 -> N-Sample Switch2/1
  Sum/1 -> Delay/1
  Unpack2/2(speed) -> MOTOR SPEED/1  "MOTOR SPEED"
  Delay2/1 -> Memory2/1
  Bus Selector1/1 -> Data Type Conversion2/1  "<Data>"
  CHINESE CORRECTION/1(Out1) -> Sum/2, Switch2/3
  Constant3/1 -> N-Sample Switch2/2
  Unpack2/1(position) -> CHINESE CORRECTION/1(position)  "MOTOR POS"
  Data Type Conversion2/1 -> Unpack2/1(Data)
  CAN Receive/2 -> Terminator1/1
  Delay/1 -> MOTOR POSITION/1
  Unpack2/3(torque) -> MOTOR TORQUE/1  "MOTOR TORQUE"

== system hip_controller_2026_02_23/Subsystem5/Right Motor Velocity1/Subsystem ==
  Motor command : Inport
  SWITCH : Inport  Port=2
  CAN Pack1 : Subsystem
  CAN Transmit1 : arduinolib/CAN Transmit  inputDataType=Raw data  BlockingMode_=on  BlockTimeout_=1  outputStatus=off  identifierType=Standard (11-bit identifier)  messageId=3  msgLength=8  remoteFrame=off
      settings: SourceProductName=Common
  Constant7 : Constant  Value=0  OutDataTypeStr=single  SampleTime=0.01
  DISABLE1 : Constant  Value=269.7/18  OutDataTypeStr=single
  Data Type Conversion3 : DataTypeConversion  OutDataTypeStr=single  SaturateOnIntegerOverflow=off  RndMeth=Floor
  Demux1 : Demux  Outputs=5
  ENABLE1 : Constant  Value=14.975  OutDataTypeStr=single
  IsNaN : RelationalOperator  Operator=isNaN  OutDataTypeStr=boolean  RndMeth=Simplest  InputSameDT=off
  N-Sample Switch4 : dspswit3/N-Sample Switch  N=15  reset=on  TriggerType=Either edge  Ts=0.01
  Rate Transition : RateTransition  OutPortSampleTime=0.01
  Subsystem2 : Subsystem
  Switch : Switch  Criteria=u2 > Threshold  SaturateOnIntegerOverflow=off  InputSameDT=off
  Switch3 : Switch  Criteria=u2 > Threshold  SaturateOnIntegerOverflow=off  InputSameDT=off
  wires:
  Demux1/4 -> CAN Pack1/4(Kd)
  Data Type Conversion3/1 -> Subsystem2/2(Velocity)
  Switch3/1 -> Subsystem2/1(Enable)
  Demux1/1 -> CAN Pack1/1(Position)
  Motor command/1 -> Data Type Conversion3/1, IsNaN/1
  Demux1/5 -> CAN Pack1/5(Torque)
  ENABLE1/1 -> Switch3/1
  Demux1/2 -> CAN Pack1/2(Velocity)
  Rate Transition/1 -> N-Sample Switch4/3
  IsNaN/1 -> Switch/2
  DISABLE1/1 -> Switch3/3
  Subsystem2/1(Enter_motor_mode) -> N-Sample Switch4/1
  Demux1/3 -> CAN Pack1/3(Kp)
  N-Sample Switch4/1 -> Demux1/1
  Switch/1 -> Rate Transition/1, Switch3/2
  CAN Pack1/1(CAN Data) -> CAN Transmit1/1
  Subsystem2/2(Velocity_value) -> N-Sample Switch4/2
  Constant7/1 -> Switch/1
  SWITCH/1 -> Switch/3

== system hip_controller_2026_02_23/Subsystem6/Left Motor Velocity/Motor Actual Position Receive ==
  SWITCH : Inport
  Bus Selector1 : BusSelector  OutputSignals=Data
  CAN Receive : arduinolib/CAN Receive  Priority=4  outputDataType=CAN Msg  identifierType=Standard (11-bit identifier)  messageId=0  msgLength=8  SampleTime=0.01  outputError=off  outputRemote=off
      settings: SourceProductName=Common
  CHINESE CORRECTION : Subsystem
  Constant1 : Constant  Value=0
  Constant3 : Constant
  Data Type Conversion2 : DataTypeConversion  OutDataTypeStr=uint16  SaturateOnIntegerOverflow=off  RndMeth=Floor
  Delay : Delay  DelayLength=1
  Delay2 : Delay
  Memory2 : Memory
  N-Sample Switch2 : dspswit3/N-Sample Switch  N=10  reset=on  TriggerType=Rising edge  Ts=0.01
  Sum : Sum  Inputs=-|+
  Switch2 : Switch  Criteria=u2 > Threshold  SaturateOnIntegerOverflow=off  InputSameDT=off
  Terminator1 : Terminator
  Unpack2 : Subsystem
  Zero-Order Hold1 : ZeroOrderHold  SampleTime=0.01
  MOTOR POSITION : Outport
  MOTOR SPEED : Outport  Port=2
  MOTOR TORQUE : Outport  Port=3
  wires:
  Switch2/1 -> Sum/1, Delay2/1
  CAN Receive/1 -> Bus Selector1/1
  SWITCH/1 -> Zero-Order Hold1/1
  N-Sample Switch2/1 -> Switch2/2
  Memory2/1 -> Switch2/1
  Constant1/1 -> N-Sample Switch2/1
  Sum/1 -> Delay/1
  Unpack2/2(speed) -> MOTOR SPEED/1  "MOTOR SPEED"
  Delay2/1 -> Memory2/1
  Bus Selector1/1 -> Data Type Conversion2/1  "<Data>"
  CHINESE CORRECTION/1(Out1) -> Sum/2, Switch2/3
  Constant3/1 -> N-Sample Switch2/2
  Unpack2/1(position) -> CHINESE CORRECTION/1(position)  "MOTOR POS"
  Data Type Conversion2/1 -> Unpack2/1(Data)
  CAN Receive/2 -> Terminator1/1
  Delay/1 -> MOTOR POSITION/1
  Unpack2/3(torque) -> MOTOR TORQUE/1  "MOTOR TORQUE"
  Zero-Order Hold1/1 -> N-Sample Switch2/3, CHINESE CORRECTION/Enable

== system hip_controller_2026_02_23/Subsystem6/Left Motor Velocity/Subsystem ==
  Motor command : Inport
  SWITCH : Inport  Port=2
  CAN Pack1 : Subsystem
  CAN Transmit1 : arduinolib/CAN Transmit  Priority=3  inputDataType=Raw data  BlockingMode_=on  BlockTimeout_=1  outputStatus=off  identifierType=Standard (11-bit identifier)  messageId=4  msgLength=8  remoteFrame=off
      settings: SourceProductName=Common
  Constant7 : Constant  Value=0  OutDataTypeStr=single  SampleTime=0.01
  DISABLE1 : Constant  Value=269.7/18  OutDataTypeStr=single
  Data Type Conversion3 : DataTypeConversion  OutDataTypeStr=single  SaturateOnIntegerOverflow=off  RndMeth=Floor
  Demux1 : Demux  Outputs=5
  ENABLE1 : Constant  Value=14.975  OutDataTypeStr=single
  IsNaN : RelationalOperator  Operator=isNaN  OutDataTypeStr=boolean  RndMeth=Simplest  InputSameDT=off
  N-Sample Switch4 : dspswit3/N-Sample Switch  N=15  reset=on  TriggerType=Either edge  Ts=0.01
  Rate Transition : RateTransition  OutPortSampleTime=0.01
  Subsystem2 : Subsystem
  Switch : Switch  Criteria=u2 > Threshold  SaturateOnIntegerOverflow=off  InputSameDT=off
  Switch3 : Switch  Criteria=u2 > Threshold  SaturateOnIntegerOverflow=off  InputSameDT=off
  wires:
  Demux1/4 -> CAN Pack1/4(Kd)
  Data Type Conversion3/1 -> Subsystem2/2(Velocity)
  Switch3/1 -> Subsystem2/1(Enable)
  Demux1/1 -> CAN Pack1/1(Position)
  Motor command/1 -> Data Type Conversion3/1, IsNaN/1
  Demux1/5 -> CAN Pack1/5(Torque)
  ENABLE1/1 -> Switch3/1
  Demux1/2 -> CAN Pack1/2(Velocity)
  Rate Transition/1 -> N-Sample Switch4/3
  IsNaN/1 -> Switch/2
  DISABLE1/1 -> Switch3/3
  Subsystem2/1(Enter_motor_mode) -> N-Sample Switch4/1
  Demux1/3 -> CAN Pack1/3(Kp)
  N-Sample Switch4/1 -> Demux1/1
  Switch/1 -> Rate Transition/1, Switch3/2
  CAN Pack1/1(CAN Data) -> CAN Transmit1/1
  Subsystem2/2(Velocity_value) -> N-Sample Switch4/2
  Constant7/1 -> Switch/1
  SWITCH/1 -> Switch/3

== system hip_controller_2026_02_23/Subsystem6/Right Motor Velocity/Motor Actual Position Receive ==
  SWITCH : Inport
  Bus Selector1 : BusSelector  OutputSignals=Data
  CAN Receive : arduinolib/CAN Receive  Priority=2  outputDataType=CAN Msg  identifierType=Standard (11-bit identifier)  messageId=0  msgLength=8  SampleTime=0.01  outputError=off  outputRemote=off
      settings: SourceProductName=Common
  CHINESE CORRECTION : Subsystem
  Constant1 : Constant  Value=0
  Constant3 : Constant
  Data Type Conversion2 : DataTypeConversion  OutDataTypeStr=uint16  SaturateOnIntegerOverflow=off  RndMeth=Floor
  Delay : Delay  DelayLength=1
  Delay2 : Delay
  Memory2 : Memory
  N-Sample Switch2 : dspswit3/N-Sample Switch  N=10  reset=on  TriggerType=Rising edge  Ts=0.01
  Sum : Sum  Inputs=-|+
  Switch2 : Switch  Criteria=u2 > Threshold  SaturateOnIntegerOverflow=off  InputSameDT=off
  Terminator1 : Terminator
  Unpack2 : Subsystem
  Zero-Order Hold1 : ZeroOrderHold  SampleTime=0.01
  MOTOR POSITION : Outport
  MOTOR SPEED : Outport  Port=2
  MOTOR TORQUE : Outport  Port=3
  wires:
  Switch2/1 -> Sum/1, Delay2/1
  CAN Receive/1 -> Bus Selector1/1
  SWITCH/1 -> Zero-Order Hold1/1
  N-Sample Switch2/1 -> Switch2/2
  Memory2/1 -> Switch2/1
  Constant1/1 -> N-Sample Switch2/1
  Sum/1 -> Delay/1
  Unpack2/2(speed) -> MOTOR SPEED/1  "MOTOR SPEED"
  Delay2/1 -> Memory2/1
  Bus Selector1/1 -> Data Type Conversion2/1  "<Data>"
  CHINESE CORRECTION/1(Out1) -> Sum/2, Switch2/3
  Constant3/1 -> N-Sample Switch2/2
  Unpack2/1(position) -> CHINESE CORRECTION/1(position)  "MOTOR POS"
  Data Type Conversion2/1 -> Unpack2/1(Data)
  CAN Receive/2 -> Terminator1/1
  Delay/1 -> MOTOR POSITION/1
  Unpack2/3(torque) -> MOTOR TORQUE/1  "MOTOR TORQUE"
  Zero-Order Hold1/1 -> N-Sample Switch2/3, CHINESE CORRECTION/Enable
